simulink model "nid_cvst_multi_instance_device"  (Simulink 10.0)
settings: Solver=FixedStepDiscrete  StartTime=0.0  StopTime=inf  RelTol=1e-3  EnableMultiTasking=on
libraries: nid_lib x5, vipsnks x3
settings Model: Creator=tchikama  LastModifiedBy=bhisma
settings DataIOCC: LimitDataPoints=on  SignalLoggingSaveFormat=ModelDataLogs  SaveOutput=off
settings OptimizationCC: ExpressionDepthLimit=2147483647  SimCompilerOptimization=on
settings DebuggingCC: SolverPrmCheckMsg=warning  FcnCallInpInsideContextMsg=warning  StateNameClashWarn=warning
settings HardwareCC: ProdIntDivRoundTo=Zero  ProdEndianess=LittleEndian  ProdHWDeviceType=Generic->32-bit x86 compatible
settings RTWCC: RTWCompilerOptimization=on
settings CodeAppCC: MaxIdLength=95
settings GRTTargetCC: GeneratePreprocessorConditionals=Disable all
settings ConfigComp: CovExternalEMLEnable=off

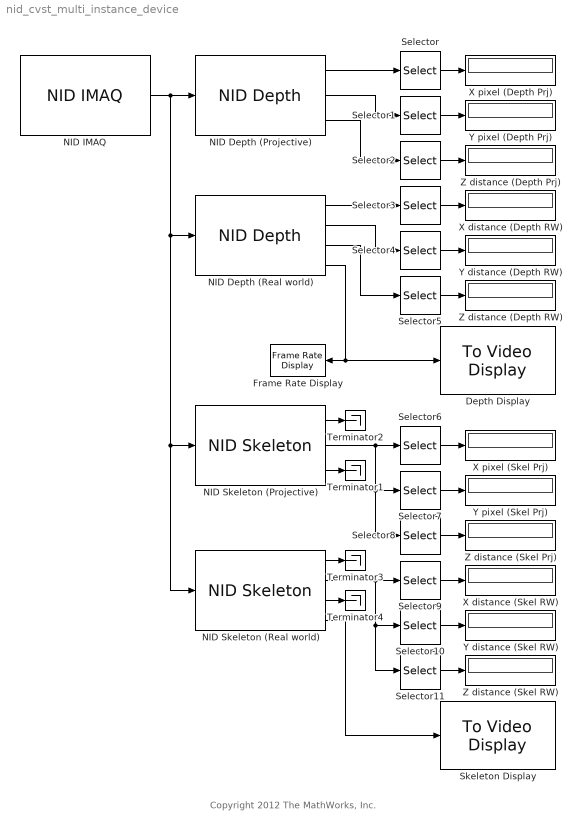
== system nid_cvst_multi_instance_device ==
  note: Copyright 2012 The MathWorks, Inc.
  Depth Display : vipsnks/To Video Display  inputType=Obsolete  imagePorts=One multidimensional signal  OutputDevice=On-screen video monitor  fullScreen=off  videoWindowX=874  videoWindowY=191  saveWindowSize=on  videoWindowWidth=440  videoWindowHeight=317  dataOrg=Column-major  openAtMdlStart=on  isWindowOpen=on
      settings: SourceProductName=Computer Vision Toolbox  SourceProductBaseCode=VP
  Frame Rate Display : vipsnks/Frame Rate Display  UpdateRate=10
      settings: SourceProductName=Computer Vision Toolbox  SourceProductBaseCode=VP
  NID Depth (Projective) : nid_lib/NID Depth  depthOutput=X/Y/Z  conv_XYZ_RW=off  viewer=off
  NID Depth (Real world) : nid_lib/NID Depth  depthOutput=X/Y/Z  conv_XYZ_RW=on  viewer=on
  NID IMAQ : nid_lib/NID IMAQ  imaq_depth=on  imaq_motion=off  imaq_image=off  view_point=off  imaq_skeleton=on  imaq_ir=off  mirror_image=off  imaq_sample_time=1/30  res_fps=VGA (640x480): 30 FPS  needPsiPose=off  angle=0  angle_read=off  near_mode=off
  NID Skeleton (Projective) : nid_lib/NID Skeleton  num_of_skeleton_tracking=2  conv_XYZ_RW=off  viewer=off
  NID Skeleton (Real world) : nid_lib/NID Skeleton  num_of_skeleton_tracking=2  conv_XYZ_RW=on  viewer=on
  Selector{,1..5} (6 alike) : Selector  NumberOfDimensions=2  IndexOptions=Index vector (dialog),Index vector (dialog)  Indices=480/2,640/2  OutputSizes=1,1
  Selector10 : Selector  NumberOfDimensions=3  IndexOptions=Index vector (dialog),Index vector (dialog),Index vector (dialog)  Indices=1,1,2  OutputSizes=1,1,1
  Selector11 : Selector  NumberOfDimensions=3  IndexOptions=Index vector (dialog),Index vector (dialog),Index vector (dialog)  Indices=1,1,3  OutputSizes=1,1,1
  Selector6 : Selector  NumberOfDimensions=3  IndexOptions=Index vector (dialog),Index vector (dialog),Index vector (dialog)  Indices=1,1,1  OutputSizes=1,1,1
  Selector7 : Selector  NumberOfDimensions=3  IndexOptions=Index vector (dialog),Index vector (dialog),Index vector (dialog)  Indices=1,1,2  OutputSizes=1,1,1
  Selector8 : Selector  NumberOfDimensions=3  IndexOptions=Index vector (dialog),Index vector (dialog),Index vector (dialog)  Indices=1,1,3  OutputSizes=1,1,1
  Selector9 : Selector  NumberOfDimensions=3  IndexOptions=Index vector (dialog),Index vector (dialog),Index vector (dialog)  Indices=1,1,1  OutputSizes=1,1,1
  Skeleton Display : vipsnks/To Video Display  inputType=Obsolete  imagePorts=One multidimensional signal  OutputDevice=On-screen video monitor  fullScreen=off  videoWindowX=873  videoWindowY=561  saveWindowSize=on  videoWindowWidth=440  videoWindowHeight=317  dataOrg=Column-major  openAtMdlStart=on  isWindowOpen=on
      settings: SourceProductName=Computer Vision Toolbox  SourceProductBaseCode=VP
  Terminator{1..4} (4 alike) : Terminator
  X distance (Depth RW) : Display
  X distance (Skel RW) : Display
  X pixel (Depth Prj) : Display
  X pixel (Skel Prj) : Display
  Y distance (Depth RW) : Display
  Y distance (Skel RW) : Display
  Y pixel (Depth Prj) : Display
  Y pixel (Skel Prj) : Display
  Z distance (Depth Prj) : Display
  Z distance (Depth RW) : Display
  Z distance (Skel Prj) : Display
  Z distance (Skel RW) : Display
  wires:
  NID IMAQ/1 -> NID Depth (Projective)/1, NID Depth (Real world)/1, NID Skeleton (Projective)/1, NID Skeleton (Real world)/1
  NID Skeleton (Projective)/2 -> Selector6/1, Selector8/1, Selector7/1
  NID Skeleton (Projective)/3 -> Terminator1/1
  NID Depth (Projective)/1 -> Selector/1
  Selector/1 -> X pixel (Depth Prj)/1
  NID Depth (Projective)/2 -> Selector1/1
  Selector1/1 -> Y pixel (Depth Prj)/1
  NID Depth (Projective)/3 -> Selector2/1
  Selector2/1 -> Z distance (Depth Prj)/1
  Selector3/1 -> X distance (Depth RW)/1
  NID Depth (Real world)/1 -> Selector3/1
  NID Depth (Real world)/2 -> Selector4/1
  NID Depth (Real world)/3 -> Selector5/1
  Selector4/1 -> Y distance (Depth RW)/1
  Selector5/1 -> Z distance (Depth RW)/1
  NID Skeleton (Projective)/1 -> Terminator2/1
  Selector6/1 -> X pixel (Skel Prj)/1
  Selector7/1 -> Y pixel (Skel Prj)/1
  Selector8/1 -> Z distance (Skel Prj)/1
  NID Depth (Real world)/4 -> Depth Display/1, Frame Rate Display/1
  NID Skeleton (Real world)/1 -> Terminator3/1
  NID Skeleton (Real world)/2 -> Selector10/1, Selector11/1, Selector9/1
  Selector9/1 -> X distance (Skel RW)/1
  Selector10/1 -> Y distance (Skel RW)/1
  NID Skeleton (Real world)/3 -> Terminator4/1
  NID Skeleton (Real world)/4 -> Skeleton Display/1
  Selector11/1 -> Z distance (Skel RW)/1
